simulink model "Engine_harness_model_power_split"  (R2021a)
settings: Solver=VariableStepAuto  StartTime=0.0  StopTime=60*10  RelTol=1e-3
PreLoadFcn:
  | Engine_harness_setup
undefined symbols (not defined in the file): engine
libraries: fl_lib x7, nesl_utility x6, sdl_lib x4
settings Model: Creator=isaacito  LastModifiedBy=isaacito
settings DataIOCC: ReturnWorkspaceOutputs=off
settings DebuggingCC: UnconnectedInputMsg=none  UnconnectedOutputMsg=none  UnconnectedLineMsg=none
settings RTWCC: DLArmComputeVersion=20.02.1
settings SimscapeCC: SimscapeLogType=all  SimscapeLogSimulationStatistics=on  SimscapeLogLimitData=off

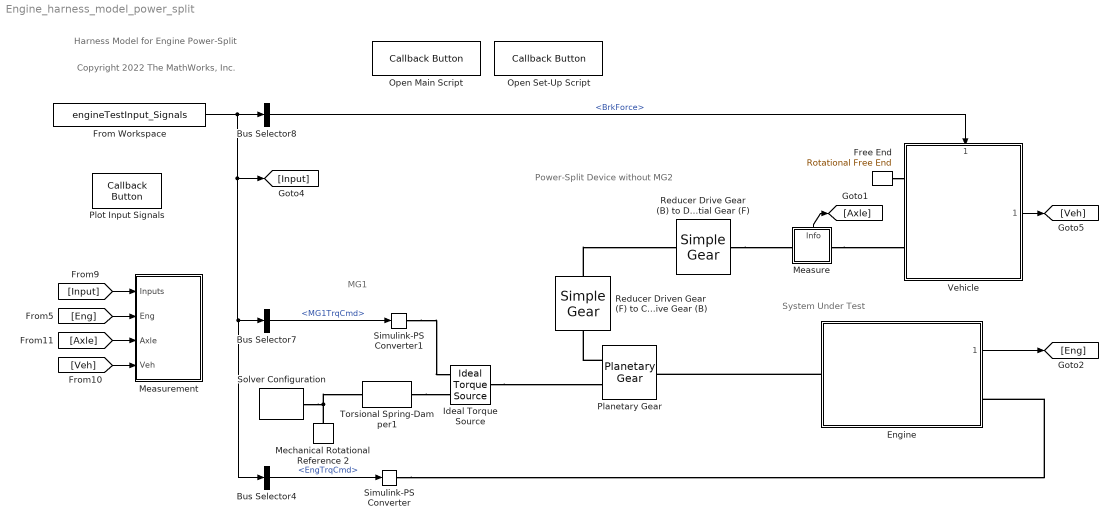
== system Engine_harness_model_power_split ==
  note: System Under Test
  note: MG1
  note: Power-Split Device without MG2
  note: Harness Model for Engine Power-Split
  note: Copyright 2022 The MathWorks, Inc.
  Bus Selector4 : BusSelector  OutputSignals=EngTrqCmd
  Bus Selector7 : BusSelector  OutputSignals=MG1TrqCmd
  Bus Selector8 : BusSelector  OutputSignals=BrkForce
  Engine : Subsystem  ReferencedSubsystem=EngineCustom_refsub
  Free End : fl_lib/Mechanical/Rotational Elements/Rotational Free End  w_specify=off  w_priority=None  w=0 rad/s  w_nominal_specify=off  w_nominal_unit=rad/s  w_nominal_value=1
      settings: SourceProductBaseCode=SS
  From Workspace : FromWorkspace  VariableName=engineTestInput_Signals  OutDataTypeStr=Bus: engineTestInput_Bus  OutputAfterFinalValue=Holding final value
      settings: AttributesFormatString=|
      | %<OutDataTypeStr>
      | Interpolate: %<Interpolate>
  Ideal Torque Source : fl_lib/Mechanical/Mechanical Sources/Ideal Torque Source
  Measure : Subsystem
      settings: PortSchema="{\"entries\":[{\"content\":{\"sides\":[{\"content\":{\"connectorIds\":[\"LConn1\"]},\"type\":\"ConnectorPlacement.EquallySpacedRectSide\",\"uuid\":\"07c3a1fd-7b75-413d-9cf1-ab8270959579\"},{\"content\":{\"connectorIds\":[\"RConn1\"],\"side\":\"RIGHT\"},\"type\":\"ConnectorPlacement.EquallySpacedRectSide\",\"uuid\":\"82fb53da-addd-4028-9f33-7d5a40e2d331\"},{\"content\":{\"connectorIds\":[\"Out1\"],\"side\":\"TOP\"},\"type\":\"ConnectorPlacement.EquallySpacedRectSide\",\"uuid\":\"88b61019-5b08-4fd4-81f8-a447296a1b8b\"}]},\"type\":\"ConnectorPlacement.EquallySpacedConnector\",\"uuid\":\"a316222e-f9ce-4776-9d48-54bd569192f1\"}],\"packageUris\":[\"http://schema.mathworks.com/mf0/Connector/R2020b\"],\"version\":\"1.0\"}"
  Measurement : Subsystem
  Mechanical Rotational Reference 2 : fl_lib/Mechanical/Rotational Elements/Mechanical Rotational Reference
  Open Main Script : CallbackButton  ButtonText=Open Main Script
      settings: ClickFcn=edit Engine_main_script
  Open Set-Up Script : CallbackButton  ButtonText=Open Set-Up Script
      settings: ClickFcn=edit Engine_harness_setup.m
  Planetary Gear : sdl_lib/Gears/Planetary Gear  rs_ratio=powerSplit.planetary_ringToSunGearRatio  friction_model=sdl.enum.gear_friction.constant  mu_visc=powerSplit.planetary_frictions_Nm_per_rpm m*N/rpm  efficiency=powerSplit.planetary_efficiencies  temperature_TLU=[280, 300, 320] K  efficiency_sp_TLU=[.95, .9, .85]  efficiency_rp_TLU=[.95, .9, .85]  pwr_thr=smoothing.planetary_meshing_loss_thresholds_W W  thermal_mass=50 J/K  T_init=300 K  model_inertia=simscape.enum.onoff.on  planet_inertia=powerSplit.planetary_planetGearInertia_kg_m2 kg*m^2
      settings: SourceProductBaseCode=LD
  Plot Input Signals : CallbackButton  ButtonText=Plot input
      settings: ClickFcn="Engine_plot_inputs_power_split(\"engineTestInput_Signals\")"
  Reducer Drive Gear (B) to Differential Gear (F) : sdl_lib/Gears/Simple Gear  ratio=powerSplit.reducer_differentialGearRatio  rotation_direction=sdl.enum.shaftOutputDirection.opposite  friction_model=sdl.enum.gear_efficiencies_load.constant  mu_visc=powerSplit.reducer_friction_Nm_per_rpm N*m/(rad/s)  T_noload=0.1 N*m  T_nom=5 N*m  efficiency_nom=0.8  efficiency=powerSplit.reducer_efficiency  temperature_TLU=[280, 300, 320] K  load_TLU=[1, 5, 10] N*m  efficiency_TLU=[.95, .9, .85]  efficiency_TLU2=[.85, .8, .75; .95, .9, .85; .85, .8, .7]  w_thr=0.01 rad/s  pwr_thr=smoothing.gear_meshing_loss_threshold_W W  thermal_mass=50 J/K  enable_faults=simscape.enum.onoff.off  efficiency_fault=0.05  external_fault=simscape.enum.onoff.off  temporal_fault=simscape.enum.onoff.off  fault_time=5 s  fault_angles=pi / 12 rad  report_fault=simscape.enum.assert.action.none  temperature_specify=off  temperature_priority=High  temperature=300 K  temperature_nominal_specify=off  temperature_nominal_unit=K  temperature_nominal_value=1
  Reducer Driven Gear (F) to Counter Drive Gear (B) : sdl_lib/Gears/Simple Gear  ratio=powerSplit.reducer_counterDriveGearRatio  rotation_direction=sdl.enum.shaftOutputDirection.opposite  friction_model=sdl.enum.gear_efficiencies_load.constant  mu_visc=powerSplit.reducer_friction_Nm_per_rpm N*m/(rad/s)  T_noload=0.1 N*m  T_nom=5 N*m  efficiency_nom=0.8  efficiency=powerSplit.reducer_efficiency  temperature_TLU=[280, 300, 320] K  load_TLU=[1, 5, 10] N*m  efficiency_TLU=[.95, .9, .85]  efficiency_TLU2=[.85, .8, .75; .95, .9, .85; .85, .8, .7]  w_thr=0.01 rad/s  pwr_thr=smoothing.gear_meshing_loss_threshold_W W  thermal_mass=50 J/K  enable_faults=simscape.enum.onoff.off  efficiency_fault=0.05  external_fault=simscape.enum.onoff.off  temporal_fault=simscape.enum.onoff.off  fault_time=5 s  fault_angles=pi / 12 rad  report_fault=simscape.enum.assert.action.none  temperature_specify=off  temperature_priority=High  temperature=300 K  temperature_nominal_specify=off  temperature_nominal_unit=K  temperature_nominal_value=1
  Simulink-PS Converter : nesl_utility/Simulink-PS Converter  PhysicalDomain=network_engine_domain  SubClassName=ps_input  LeftPortType=input  RightPortType=output  PseudoPeriodic=off  Frequencies=[]  NoiseDistribution=none  NoiseParameters=[]  Unit=N*m  AffineConversion=off  FilteringAndDerivatives=provide  SimscapeFilterOrder=1  InputFilterTimeConstant=0.001  UdotUserProvided=0
      settings: SourceProductBaseCode=SS,PW,VE
  Simulink-PS Converter1 : nesl_utility/Simulink-PS Converter  PhysicalDomain=network_engine_domain  SubClassName=ps_input  LeftPortType=input  RightPortType=output  PseudoPeriodic=off  Frequencies=[]  NoiseDistribution=none  NoiseParameters=[]  Unit=N*m  AffineConversion=off  FilteringAndDerivatives=filter  SimscapeFilterOrder=1  InputFilterTimeConstant=0.001  UdotUserProvided=0
      settings: SourceProductBaseCode=SS,PW,VE
  Solver Configuration : nesl_utility/Solver Configuration  PhysicalDomain=network_engine_domain  SubClassName=solver  LeftPortType=input  RightPortType=generic  Tones=[]  Harmonics=[]  SimulateNoise=off  Profile=off  UseLocalSampling=off  EnableSwitchedLinearOptims=on  FrequencyDomain=off  UseCCode=off  RelTol=0.001  AbsTol=0.001  MinStep=1e-09  ToWorkspace=off  RevertToSquareIcSolve=off  NumHomotopyIterations=100  PhasorMode=off  PhasorModeNumHarmonics=1  DoDC=off  ResidualTolerance=1e-09  UseLocalSolver=off  LocalSolverChoice=NE_BACKWARD_EULER_ADVANCER  LocalSolverSampleTime=0.001  DoFixedCost=off  MaxNonlinIter=3  MaxModeIter=2  ComputeImpulses=off  ImpulseIterations=2  LinearAlgebra=auto  EquationFormulation=NE_TIME_EF  DelaysMemoryBudget=1024  AutomaticFiltering=on  FilteringTimeConstant=0.001  PartitionStorageMethod=AS_NEEDED  PartitionMemoryBudget=1024  PartitionMethod=ROBUST
      settings: AttributesFormatString=Local solver: %<UseLocalSolver>  SourceProductBaseCode=SS,PW,VE
  Torsional Spring-Damper1 : sdl_lib/Couplings & Drives/Torsional Spring-Damper  k=engine.dampSpringStiffness_Nm_per_rad N*m/rad  mu_visc=engine.dampSpringFriction_Nm_per_rpm m*N/rpm  trq_coulomb=0 N*m  static_kinetic_ratio=1.1  w_tol=smoothing.engine_dampSpringVelTol_rpm rpm  model_hardstop=0  upper_bound=10 deg  lower_bound=-10 deg  k_endstop=1e6 N*m/rad  D_endstop=10 N*m/(rad/s)  hardstop_model=1  transition=0.001 rad  x0=0 deg
      settings: SourceProductBaseCode=LD  InternalSimscapePortConfiguration="{\"Bottom\":[],\"Left\":[{\"id\":\"R\",\"label\":\"R\",\"type\":\"foundation.mechanical.rotational.rotational\"}],\"Right\":[{\"id\":\"C\",\"label\":\"C\",\"type\":\"foundation.mechanical.rotational.rotational\"}],\"Top\":[]}"
  Vehicle : Subsystem  ReferencedSubsystem=VehicleForTest2_refsub
      settings: PortSchema="{\"entries\":[{\"content\":{\"sides\":[{\"content\":{\"connectorIds\":[\"LConn1\",\"LConn2\"]},\"type\":\"ConnectorPlacement.EquallySpacedRectSide\",\"uuid\":\"eee003cc-6e5e-4208-ae9b-9bf73ca57d34\"},{\"content\":{\"connectorIds\":[\"Out1\"],\"side\":\"RIGHT\"},\"type\":\"ConnectorPlacement.EquallySpacedRectSide\",\"uuid\":\"d6e495c3-442b-470a-90f0-05b37cdcae3e\"},{\"content\":{\"connectorIds\":[\"In1\"],\"side\":\"TOP\"},\"type\":\"ConnectorPlacement.EquallySpacedRectSide\",\"uuid\":\"ffec2806-13d3-440e-b6db-b8cc25f5bd66\"}]},\"type\":\"ConnectorPlacement.EquallySpacedConnector\",\"uuid\":\"c9cc6dfd-d4e7-4457-9549-27666fa7b630\"}],\"packageUris\":[\"http://schema.mathworks.com/mf0/Connector/R2020b\"],\"version\":\"1.0\"}"
  wires:
  Measure/1(Info) -> [Axle]
  From Workspace/1 -> Bus Selector4/1, Bus Selector7/1, [Input], Bus Selector8/1
  Engine/1 -> [Eng]
  Bus Selector4/1 -> Simulink-PS Converter/1  "<EngTrqCmd>"
  Bus Selector7/1 -> Simulink-PS Converter1/1  "<MG1TrqCmd>"
  Bus Selector8/1 -> Vehicle/1  "<BrkForce>"
  Vehicle/1 -> [Veh]
  [Eng] -> Measurement/2(Eng)
  [Input] -> Measurement/1(Inputs)
  [Axle] -> Measurement/3(Axle)
  [Veh] -> Measurement/4(Veh)
  connections:
  Reducer Drive Gear (B) to Differential Gear (F)/LConn1 -- Measure/LConn1
  Ideal Torque Source/LConn1 -- Planetary Gear/RConn2
  Torsional Spring-Damper1/RConn1 -- Ideal Torque Source/RConn2
  Mechanical Rotational Reference 2/LConn1 -- Solver Configuration/RConn1 -- Torsional Spring-Damper1/LConn1
  Simulink-PS Converter1/RConn1 -- Ideal Torque Source/RConn1
  Planetary Gear/RConn1 -- Reducer Driven Gear (F) to Counter Drive Gear (B)/LConn1
  Reducer Driven Gear (F) to Counter Drive Gear (B)/RConn1 -- Reducer Drive Gear (B) to Differential Gear (F)/RConn1
  Measure/RConn1 -- Vehicle/LConn2
  Engine/LConn1 -- Planetary Gear/LConn1
  Simulink-PS Converter/RConn1 -- Engine/RConn1
  Free End/LConn1 -- Vehicle/LConn1

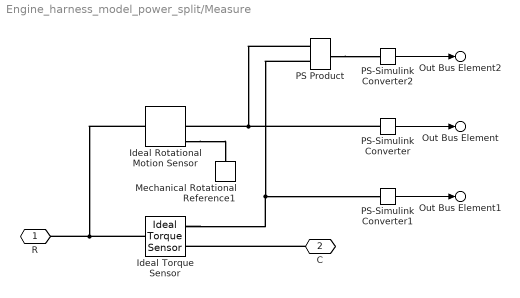
== system Engine_harness_model_power_split/Measure ==
  Ideal Rotational Motion Sensor : fl_lib/Mechanical/Mechanical Sensors/Ideal Rotational Motion Sensor  wrap_angle=simscape.enum.onoff.off  offset=0 rad
      settings: SourceProductBaseCode=PW,SS,VE
  Ideal Torque Sensor : fl_lib/Mechanical/Mechanical Sensors/Ideal Torque Sensor
      settings: SourceProductBaseCode=PW,SS,VE
  Mechanical Rotational Reference1 : fl_lib/Mechanical/Rotational Elements/Mechanical Rotational Reference
      settings: SourceProductBaseCode=PW,SS,VE
  PS Product : fl_lib/Physical Signals/Functions/PS Product
  PS-Simulink Converter : nesl_utility/PS-Simulink Converter  PhysicalDomain=network_engine_domain  SubClassName=ps_output  LeftPortType=input  RightPortType=output  PseudoPeriodic=off  Frequencies=[]  Unit=rpm  AffineConversion=off
      settings: SourceProductBaseCode=SS,PW,VE
  PS-Simulink Converter1 : nesl_utility/PS-Simulink Converter  PhysicalDomain=network_engine_domain  SubClassName=ps_output  LeftPortType=input  RightPortType=output  PseudoPeriodic=off  Frequencies=[]  Unit=N*m  AffineConversion=off
      settings: SourceProductBaseCode=SS,PW,VE
  PS-Simulink Converter2 : nesl_utility/PS-Simulink Converter  PhysicalDomain=network_engine_domain  SubClassName=ps_output  LeftPortType=input  RightPortType=output  PseudoPeriodic=off  Frequencies=[]  Unit=kW  AffineConversion=off
      settings: SourceProductBaseCode=SS,PW,VE
  R : PMIOPort  Side=Left
  C : PMIOPort  Port=2  Side=Right
  Out Bus Element : Outport  PortName=Info  Element=AxleSpd
  Out Bus Element1 : Outport  PortName=Info  Element=AxleTrq
  Out Bus Element2 : Outport  PortName=Info  Element=AxlePwr
  wires:
  PS-Simulink Converter/1 -> Out Bus Element/1
  PS-Simulink Converter1/1 -> Out Bus Element1/1
  PS-Simulink Converter2/1 -> Out Bus Element2/1
  connections:
  PS-Simulink Converter/LConn1 -- PS Product/LConn1 -- Ideal Rotational Motion Sensor/RConn2
  Ideal Rotational Motion Sensor/RConn1 -- Mechanical Rotational Reference1/LConn1
  Ideal Torque Sensor/RConn2 -- PS Product/LConn2 -- PS-Simulink Converter1/LConn1
  Ideal Torque Sensor/LConn1 -- R/RConn1 -- Ideal Rotational Motion Sensor/LConn1
  C/RConn1 -- Ideal Torque Sensor/RConn1
  PS Product/RConn1 -- PS-Simulink Converter2/LConn1

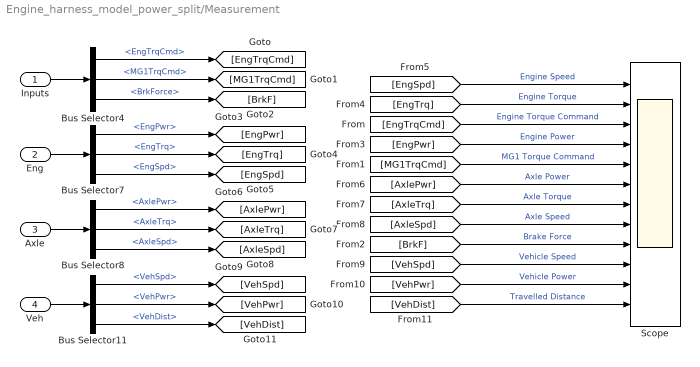
== system Engine_harness_model_power_split/Measurement ==
  Inputs : Inport
  Eng : Inport  Port=2
  Axle : Inport  Port=3
  Veh : Inport  Port=4
  Bus Selector11 : BusSelector  OutputSignals=VehSpd,VehPwr,VehDist
  Bus Selector4 : BusSelector  OutputSignals=EngTrqCmd,MG1TrqCmd,BrkForce
  Bus Selector7 : BusSelector  OutputSignals=EngPwr,EngTrq,EngSpd
  Bus Selector8 : BusSelector  OutputSignals=AxlePwr,AxleTrq,AxleSpd
  Scope : Scope  NumInputPorts=12
  wires:
  Inputs/1 -> Bus Selector4/1
  Bus Selector4/1 -> [EngTrqCmd]  "<EngTrqCmd>"
  Bus Selector4/3 -> [BrkF]  "<BrkForce>"
  Bus Selector4/2 -> [MG1TrqCmd]  "<MG1TrqCmd>"
  Eng/1 -> Bus Selector7/1
  Bus Selector7/1 -> [EngPwr]  "<EngPwr>"
  Bus Selector7/2 -> [EngTrq]  "<EngTrq>"
  Bus Selector7/3 -> [EngSpd]  "<EngSpd>"
  Bus Selector8/3 -> [AxleSpd]  "<AxleSpd>"
  Bus Selector8/1 -> [AxlePwr]  "<AxlePwr>"
  Bus Selector8/2 -> [AxleTrq]  "<AxleTrq>"
  Axle/1 -> Bus Selector8/1
  Bus Selector11/1 -> [VehSpd]  "<VehSpd>"
  Bus Selector11/2 -> [VehPwr]  "<VehPwr>"
  Bus Selector11/3 -> [VehDist]  "<VehDist>"
  Veh/1 -> Bus Selector11/1
  [EngSpd] -> Scope/1  "Engine Speed"
  [EngTrq] -> Scope/2  "Engine Torque"
  [EngTrqCmd] -> Scope/3  "Engine Torque Command"
  [EngPwr] -> Scope/4  "Engine Power"
  [MG1TrqCmd] -> Scope/5  "MG1 Torque Command"
  [AxlePwr] -> Scope/6  "Axle Power"
  [AxleTrq] -> Scope/7  "Axle Torque"
  [AxleSpd] -> Scope/8  "Axle Speed"
  [BrkF] -> Scope/9  "Brake Force"
  [VehSpd] -> Scope/10  "Vehicle Speed"
  [VehPwr] -> Scope/11  "Vehicle Power"
  [VehDist] -> Scope/12  "Travelled Distance"
